simulink model "S13_PASD_as3"  (R2020a)
settings: Solver=VariableStepAuto  StartTime=0.0  StopTime=0.5  RelTol=1e-3
libraries: powerlib x32, cstblocks x1, simulink x1
settings Model: Creator=HP  LastModifiedBy=qm_shail_hash_98
settings DataIOCC: SaveFormat=StructureWithTime  InspectSignalLogs=on  ReturnWorkspaceOutputs=off

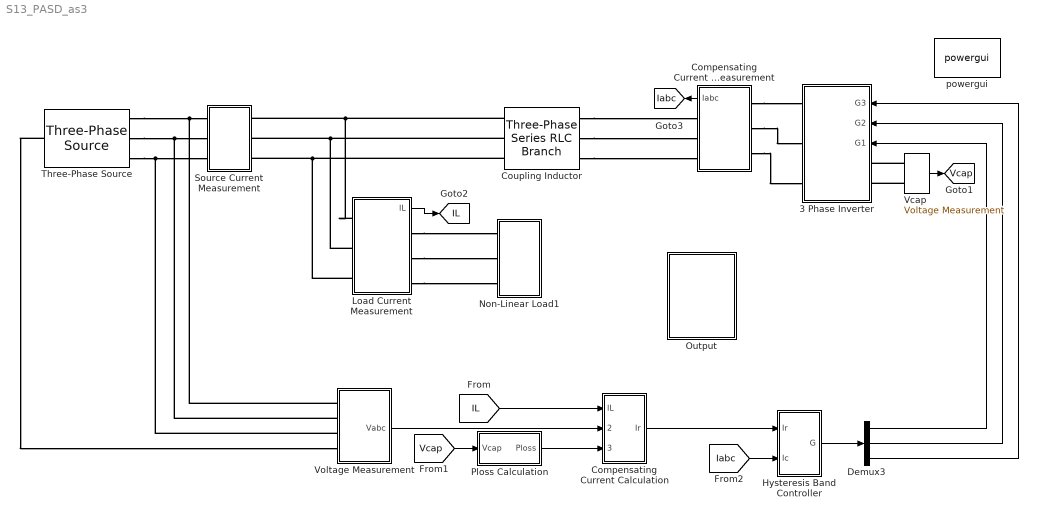
== system S13_PASD_as3 ==
  3 Phase Inverter : Subsystem
  Compensating Current Calculation : Subsystem
  Compensating Current Measurement : Subsystem
  Coupling Inductor : powerlib/Elements/Three-Phase Series RLC Branch  LConnTagsString=A|B|C  RConnTagsString=A|B|C  BranchType=RL  Resistance=0.0001  Inductance=0.0004  Capacitance=1e-6  Measurements=None
  Demux3 : Demux  Outputs=3
  Hysteresis Band Controller : Subsystem
  Load Current Measurement : Subsystem
  "Non-Linear Load1 " : Subsystem
  Output : Subsystem
  Ploss Calculation : Subsystem
  Source Current Measurement : Subsystem
  Three-Phase Source : powerlib/Electrical Sources/Three-Phase Source  InternalConnection=Yn  VoltagePhases=off  Voltage=400  PhaseAngle=0  Voltage_phases=[25e3 25e3 25e3]/sqrt(3)  PhaseAngles_phases=[0 -120 +120]  Frequency=50  NonIdealSource=on  SpecifyImpedance=on  Resistance=0.8929  Inductance=16.58e-3  ShortCircuitLevel=100e6  BaseVoltage=40.83  XRratio=10  BusType=swing  Pref=0  Qref=0  Prefabc=[10e3, 10e3, 10e3]  Qrefabc=[0, 0, 0]  Qmin=-inf  Qmax=inf
  Vcap : powerlib/Measurements/Voltage Measurement  PhasorSimulation=off  OutputType=Complex  PSBequivalent=0
  Voltage Measurement : Subsystem
  powergui : powerlib/powergui  Priority=1  SimulationMode=Discrete  SampleTime=5e-7  frequency=60  Iterations=50  frequencyindice=50  Pbase=100e6  ErrMax=1e-4  UnitsV=kV  UnitsW=MW  buscounter=0  FunctionMessages=off  echomessages=off  EnableUseOfTLC=off  CurrentSourceSwitches=off  DisableSnubberDevices=off  DisableRonSwitches=off  DisableVfSwitches=off  DisplayEquations=off  AutomaticDiscreteSolvers=off  SolverType=Backward Euler  Interpol=off  ExternalGateDelay=off  methode=off  Ts=0  x0status=blocks  SPID=off  SwTol=0  HookPort=off  NonlinearTolerance=1e-4  nMaxIteration=100  ContinueOnMaxIteration=off  RestoreLinks=warning  ResistiveCurrentMeasurement=off  Frange=[0:2:500]  Ylog=off  Xlog=on  ShowGrid=off  save=off  variable=ZData  structure=IS  ZoomFFT=off  StartTime=0.3  cycles=5  DisplayStyle=1  fundamental=50  FreqAxis=off  MaxFrequency=1000  frequencyindicesteady=1  RmsSteady=1  display=off
  tag scope: IL=global, Iabc=global, Vcap=global
  wires:
  Load Current Measurement/1(IL) -> [IL]
  [IL] -> Compensating Current Calculation/1(IL)
  Voltage Measurement/1(Vabc) -> Compensating Current Calculation/2(Vabc)
  Ploss Calculation/1(Ploss) -> Compensating Current Calculation/3(Ploss)
  [Vcap] -> Ploss Calculation/1(Vcap)
  Vcap/1 -> [Vcap]
  Hysteresis Band Controller/1(G) -> Demux3/1
  Demux3/2 -> 3 Phase Inverter/2(G2)
  Compensating Current Calculation/1(Ir) -> Hysteresis Band Controller/1(Ir)
  Compensating Current Measurement/1(Iabc) -> [Iabc]
  [Iabc] -> Hysteresis Band Controller/2(Ic)
  Demux3/1 -> 3 Phase Inverter/3(G1)
  Demux3/3 -> 3 Phase Inverter/1(G3)
  connections:
  Three-Phase Source/RConn1 -- Voltage Measurement/LConn1 -- Source Current Measurement/LConn1
  Three-Phase Source/RConn2 -- Voltage Measurement/LConn2 -- Source Current Measurement/LConn2
  Three-Phase Source/RConn3 -- Voltage Measurement/LConn3 -- Source Current Measurement/LConn3
  Three-Phase Source/LConn1 -- Voltage Measurement/LConn4
  Load Current Measurement/LConn3 -- Coupling Inductor/LConn3 -- Source Current Measurement/RConn3
  Load Current Measurement/LConn1 -- Source Current Measurement/RConn1 -- Coupling Inductor/LConn1
  Load Current Measurement/LConn2 -- Coupling Inductor/LConn2 -- Source Current Measurement/RConn2
  Vcap/LConn2 -- 3 Phase Inverter/LConn2
  Load Current Measurement/RConn1 -- "Non-Linear Load1 "/LConn1
  Load Current Measurement/RConn2 -- "Non-Linear Load1 "/LConn2
  Load Current Measurement/RConn3 -- "Non-Linear Load1 "/LConn3
  Vcap/LConn1 -- 3 Phase Inverter/LConn1
  Compensating Current Measurement/LConn1 -- 3 Phase Inverter/RConn1
  Compensating Current Measurement/LConn2 -- 3 Phase Inverter/RConn2
  Compensating Current Measurement/LConn3 -- 3 Phase Inverter/RConn3
  Coupling Inductor/RConn1 -- Compensating Current Measurement/RConn1
  Coupling Inductor/RConn2 -- Compensating Current Measurement/RConn2
  Coupling Inductor/RConn3 -- Compensating Current Measurement/RConn3

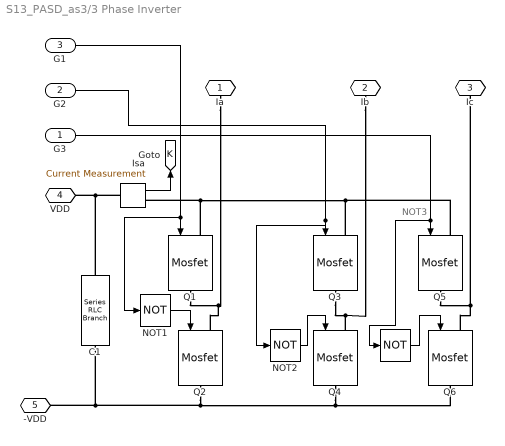
== system S13_PASD_as3/3 Phase Inverter ==
  note: NOT3
  G3 : Inport
  G2 : Inport  Port=2
  G1 : Inport  Port=3
  " " : Logic  Operator=NOT  AllPortsSameDT=off  OutDataTypeStr=boolean
  C1 : powerlib/Elements/Series RLC Branch  LConnTagsString=__new0  RConnTagsString=__new0  BranchType=C  Resistance=1  Inductance=1e-3  SetiL0=off  InitialCurrent=0  Capacitance=500e-6  Setx0=off  InitialVoltage=700  Measurements=None
  Isa : powerlib/Measurements/Current Measurement  PhasorSimulation=off  OutputType=Complex  PSBequivalent=0
  NOT1 : Logic  Operator=NOT  AllPortsSameDT=off  OutDataTypeStr=boolean
  NOT2 : Logic  Operator=NOT  AllPortsSameDT=off  OutDataTypeStr=boolean
  Q{1..6} (6 alike) : powerlib/Power Electronics/Mosfet  Ron=0.01  Lon=0  Rd=0.01  Vfd=0  IC=0  Rs=1e10  Cs=inf  Measurements=off
  Ia : PMIOPort  Side=Right
  Ib : PMIOPort  Port=2  Side=Right
  Ic : PMIOPort  Port=3  Side=Right
  VDD : PMIOPort  Port=4  Side=Left
  -VDD : PMIOPort  Port=5  Side=Left
  tag scope: K=global
  wires:
  NOT1/1 -> Q2/1
  NOT2/1 -> Q4/1
  " "/1 -> Q6/1
  G1/1 -> NOT1/1, Q1/1
  G2/1 -> Q3/1, NOT2/1
  G3/1 -> Q5/1, " "/1
  Isa/1 -> [K]
  connections:
  Q1/RConn1 -- Ia/RConn1 -- Q2/LConn1
  Isa/LConn1 -- VDD/RConn1 -- C1/LConn1
  Q3/RConn1 -- Ib/RConn1 -- Q4/LConn1
  Q6/LConn1 -- Ic/RConn1 -- Q5/RConn1
  Q1/LConn1 -- Isa/RConn1 -- Q5/LConn1 -- Q3/LConn1
  Q2/RConn1 -- C1/RConn1 -- -VDD/RConn1 -- Q4/RConn1 -- Q6/RConn1

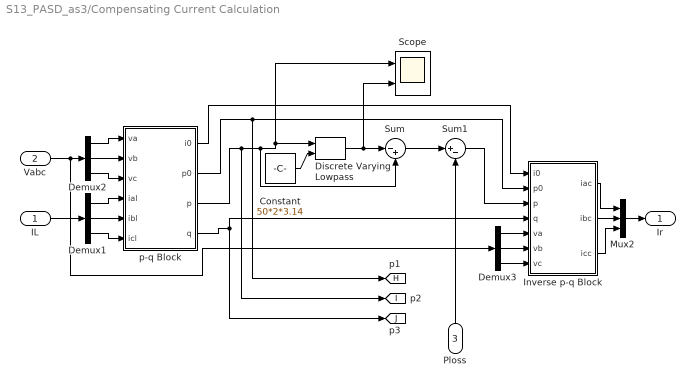
== system S13_PASD_as3/Compensating Current Calculation ==
  IL : Inport
  Vabc : Inport  Port=2
  Ploss : Inport  Port=3
  Constant : Constant  Value=50*2*3.14
  Demux1 : Demux  Outputs=3
  Demux2 : Demux  Outputs=3
  Demux3 : Demux  Outputs=3
  Discrete Varying Lowpass : cstblocks/Linear Parameter Varying/Discrete Varying Lowpass  N=3  w0=0  Ts=1e-3
      settings: SourceProductBaseCode=CT
  Inverse p-q Block : MATLAB Function  TreatAsAtomicUnit=on
  Mux2 : Mux  Inputs=3
  Scope : Scope  NumInputPorts=2
  Sum : Sum  Inputs=|-+
  Sum1 : Sum  Inputs=|+-
  p-q Block : MATLAB Function  TreatAsAtomicUnit=on
  Ir : Outport
  tag scope: H=global, I=global, J=global
  wires:
  Inverse p-q Block/3(icc) -> Mux2/3
  IL/1 -> Demux1/1
  Demux1/2 -> p-q Block/5(ibl)
  Mux2/1 -> Ir/1
  Inverse p-q Block/1(iac) -> Mux2/1
  Demux1/1 -> p-q Block/4(ial)
  Inverse p-q Block/2(ibc) -> Mux2/2
  p-q Block/1(i0) -> Inverse p-q Block/1(i0)
  p-q Block/3(p) -> [I], Scope/1, Discrete Varying Lowpass/1, Sum/2
  Ploss/1 -> Sum1/2
  Discrete Varying Lowpass/1 -> Scope/2, Sum/1
  Sum/1 -> Sum1/1
  Sum1/1 -> Inverse p-q Block/3(p)
  p-q Block/4(q) -> [J], Inverse p-q Block/4(q)
  Demux1/3 -> p-q Block/6(icl)
  p-q Block/2(p0) -> [H], Inverse p-q Block/2(p0)
  Demux2/3 -> p-q Block/3(vc)
  Demux2/2 -> p-q Block/2(vb)
  Demux2/1 -> p-q Block/1(va)
  Vabc/1 -> Demux3/1, Demux2/1
  Demux3/1 -> Inverse p-q Block/5(va)
  Demux3/2 -> Inverse p-q Block/6(vb)
  Demux3/3 -> Inverse p-q Block/7(vc)
  Constant/1 -> Discrete Varying Lowpass/2

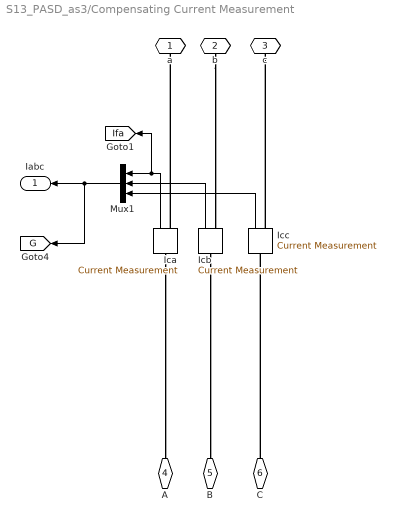
== system S13_PASD_as3/Compensating Current Measurement ==
  Ica : powerlib/Measurements/Current Measurement  PhasorSimulation=off  OutputType=Complex  PSBequivalent=0
  Icb : powerlib/Measurements/Current Measurement  PhasorSimulation=off  OutputType=Complex  PSBequivalent=0
  Icc : powerlib/Measurements/Current Measurement  PhasorSimulation=off  OutputType=Complex  PSBequivalent=0
  Mux1 : Mux  Inputs=3
  a : PMIOPort  Side=Right
  b : PMIOPort  Port=2  Side=Right
  c : PMIOPort  Port=3  Side=Right
  A : PMIOPort  Port=4  Side=Left
  B : PMIOPort  Port=5  Side=Left
  C : PMIOPort  Port=6  Side=Left
  Iabc : Outport
  tag scope: G=global, Ifa=global
  wires:
  Mux1/1 -> [G], Iabc/1
  Ica/1 -> Mux1/1, [Ifa]
  Icc/1 -> Mux1/3
  Icb/1 -> Mux1/2
  connections:
  b/RConn1 -- Icb/RConn1
  Ica/RConn1 -- a/RConn1
  Icc/RConn1 -- c/RConn1
  C/RConn1 -- Icc/LConn1
  Ica/LConn1 -- A/RConn1
  Icb/LConn1 -- B/RConn1

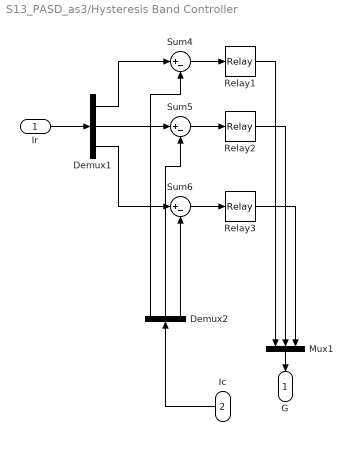
== system S13_PASD_as3/Hysteresis Band Controller ==
  Ir : Inport
  Ic : Inport  Port=2
  Demux1 : Demux  Outputs=3
  Demux2 : Demux  Outputs=3
  Mux1 : Mux  Inputs=3
  Relay1 : Relay  OnSwitchValue=0.0001  OffSwitchValue=-0.0001  ZeroCross=off
  Relay2 : Relay  OnSwitchValue=0.0001  OffSwitchValue=-0.0001  ZeroCross=off
  Relay3 : Relay  OnSwitchValue=0.0001  OffSwitchValue=-0.0001  ZeroCross=off
  Sum4 : Sum  Inputs=|+-
  Sum5 : Sum  Inputs=|+-
  Sum6 : Sum  Inputs=|+-
  G : Outport
  wires:
  Relay3/1 -> Mux1/3
  Relay1/1 -> Mux1/1
  Relay2/1 -> Mux1/2
  Demux2/2 -> Sum5/2
  Demux1/2 -> Sum5/1
  Sum6/1 -> Relay3/1
  Demux1/1 -> Sum4/1
  Demux1/3 -> Sum6/1
  Demux2/3 -> Sum6/2
  Sum5/1 -> Relay2/1
  Demux2/1 -> Sum4/2
  Sum4/1 -> Relay1/1
  Mux1/1 -> G/1
  Ir/1 -> Demux1/1
  Ic/1 -> Demux2/1

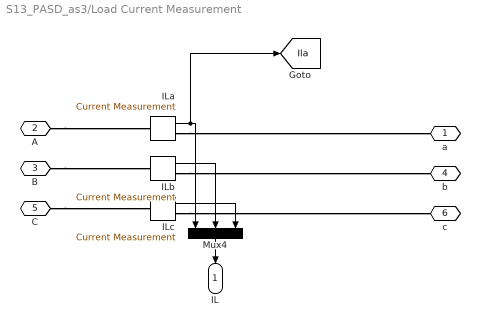
== system S13_PASD_as3/Load Current Measurement ==
  ILa : powerlib/Measurements/Current Measurement  PhasorSimulation=off  OutputType=Complex  PSBequivalent=0
  ILb : powerlib/Measurements/Current Measurement  PhasorSimulation=off  OutputType=Complex  PSBequivalent=0
  ILc : powerlib/Measurements/Current Measurement  PhasorSimulation=off  OutputType=Complex  PSBequivalent=0
  Mux4 : Mux  Inputs=3
  a : PMIOPort  Side=Right
  A : PMIOPort  Port=2  Side=Left
  B : PMIOPort  Port=3  Side=Left
  b : PMIOPort  Port=4  Side=Right
  C : PMIOPort  Port=5  Side=Left
  c : PMIOPort  Port=6  Side=Right
  IL : Outport
  tag scope: Ila=global
  wires:
  Mux4/1 -> IL/1
  ILa/1 -> [Ila], Mux4/1
  ILc/1 -> Mux4/3
  ILb/1 -> Mux4/2
  connections:
  ILb/RConn1 -- b/RConn1
  ILa/RConn1 -- a/RConn1
  ILc/RConn1 -- c/RConn1
  A/RConn1 -- ILa/LConn1
  C/RConn1 -- ILc/LConn1
  B/RConn1 -- ILb/LConn1

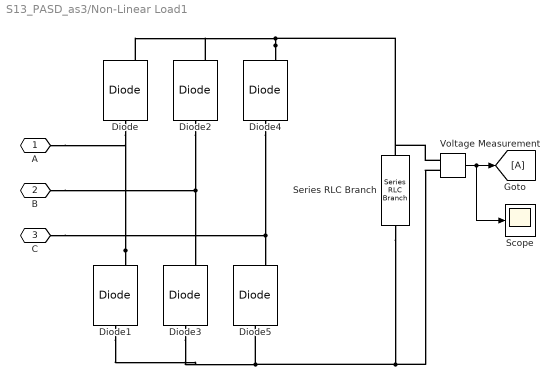
== system S13_PASD_as3/Non-Linear Load1  ==
  Diode{,1..5} (6 alike) : powerlib/Power Electronics/Diode  Ron=0.001  Lon=0  Vf=0.8  IC=0  UseSnubber=0  Rs=500  Cs=250e-9  Measurements=on
  Scope : Scope
  Series RLC Branch : powerlib/Elements/Series RLC Branch  LConnTagsString=__new0  RConnTagsString=__new0  BranchType=RL  Resistance=40  Inductance=0.5  SetiL0=off  InitialCurrent=0  Capacitance=1e-6  Setx0=off  InitialVoltage=0  Measurements=None
  Voltage Measurement : powerlib/Measurements/Voltage Measurement  PhasorSimulation=off  OutputType=Complex  PSBequivalent=0
  A : PMIOPort  Side=Left
  B : PMIOPort  Port=2  Side=Left
  C : PMIOPort  Port=3  Side=Left
  wires:
  Voltage Measurement/1 -> Scope/1, [A]
  connections:
  Diode4/RConn1 -- Voltage Measurement/LConn1 -- Series RLC Branch/LConn1 -- Diode/RConn1 -- Diode2/RConn1
  Series RLC Branch/RConn1 -- Diode5/LConn1 -- Diode1/LConn1 -- Diode3/LConn1 -- Voltage Measurement/LConn2
  Diode1/RConn1 -- Diode/LConn1 -- A/RConn1
  Diode2/LConn1 -- Diode3/RConn1 -- B/RConn1
  Diode4/LConn1 -- C/RConn1 -- Diode5/RConn1

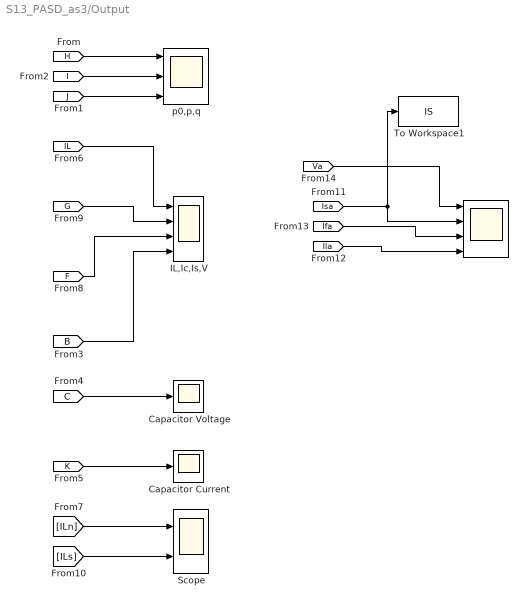
== system S13_PASD_as3/Output ==
  " " : Scope  NumInputPorts=4
  Capacitor Current : Scope
  Capacitor Voltage : Scope
  IL,Ic,Is,V : Scope  NumInputPorts=4
  Scope : Scope  NumInputPorts=2
  To Workspace1 : ToWorkspace  VariableName=IS  SaveFormat=Structure With Time  SampleTime=-1
  p0,p,q : Scope  NumInputPorts=3
  wires:
  [C] -> Capacitor Voltage/1
  [F] -> IL,Ic,Is,V/3
  [IL] -> IL,Ic,Is,V/1
  [B] -> IL,Ic,Is,V/4
  [G] -> IL,Ic,Is,V/2
  [H] -> p0,p,q/1
  [I] -> p0,p,q/2
  [J] -> p0,p,q/3
  [K] -> Capacitor Current/1
  [ILn] -> Scope/1
  [ILs] -> Scope/2
  [Ila] -> " "/4
  [Ifa] -> " "/3
  [Isa] -> To Workspace1/1, " "/2
  [Va] -> " "/1

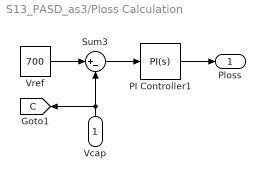
== system S13_PASD_as3/Ploss Calculation ==
  Vcap : Inport
  PI Controller1 : simulink/Continuous/PID Controller  Controller=PI  Form=Parallel  TimeDomain=Continuous-time  UseExternalTs=off  SampleTime=-1  IntegratorMethod=Forward Euler  FilterMethod=Forward Euler  ControllerParametersSource=internal  P=31.1  I=5  D=0  UseFilter=on  N=100  TunerSelectOption=Frequency Response Based  ZeroCross=off  InitialConditionSource=internal  InitialConditionForIntegrator=0  InitialConditionForFilter=0  DifferentiatorICPrevScaledInput=0  ExternalReset=none  TrackingMode=off  Kt=1  LimitOutput=off  UpperSaturationLimit=inf  LowerSaturationLimit=-inf  LinearizeAsGain=off  AntiWindupMode=none  Kb=1  POutMin=[]  POutMax=[]  IOutMin=[]  IOutMax=[]  DOutMin=[]  DOutMax=[]  NOutMin=[]  NOutMax=[]  SumOutMin=[]  SumOutMax=[]  SaturationOutMin=[]  SaturationOutMax=[]  PParamMin=[]  PParamMax=[]  IParamMin=[]  IParamMax=[]  DParamMin=[]  DParamMax=[]  NParamMin=[]  NParamMax=[]  KbParamMin=[]  KbParamMax=[]  KtParamMin=[]  KtParamMax=[]  KbOutMin=[]  KbOutMax=[]  KtOutMin=[]  KtOutMax=[]  IntegratorOutMin=[]  IntegratorOutMax=[]  FilterOutMin=[]  FilterOutMax=[]  SumI1OutMin=[]  SumI1OutMax=[]  SumI2OutMin=[]  SumI2OutMax=[]  SumI3OutMin=[]  SumI3OutMax=[]  SumI4OutMin=[]  SumI4OutMax=[]  SumDOutMin=[]  SumDOutMax=[]  DifferentiatorOutMin=[]  DifferentiatorOutMax=[]  FilterDiffOutCoefMin=[]  FilterDiffOutCoefMax=[]  ReciprocalOutMin=[]  ReciprocalOutMax=[]  SumDenOutMin=[]  SumDenOutMax=[]  SumNumOutMin=[]  SumNumOutMax=[]  DivideOutMin=[]  DivideOutMax=[]  UdiffTsProdOutMin=[]  UdiffTsProdOutMax=[]  NTsProdOutMin=[]  NTsProdOutMax=[]  UintegralTsProdOutMin=[]  UintegralTsProdOutMax=[]  UngainTsProdOutMin=[]  UngainTsProdOutMax=[]  IntegratorContinuousStateAttributes=''  IntegratorStateMustResolveToSignalObject=off  IntegratorRTWStateStorageClass=Auto  FilterContinuousStateAttributes=''  FilterStateMustResolveToSignalObject=off  FilterRTWStateStorageClass=Auto  ParallelPVariant=InternalParameters  IdealPVariant=Disabled  IVariant=InternalParameters  DVariant=Disabled  IntegratorVariant=Continuous  SatVariant=Disabled  AWVariant=Passthrough  PCopyVariant=Disabled  TRVariant=Disabled  FdbkBlocksVariant=Forward  IdealPFdbkVariant=Disabled  SatFdbkVariant=Disabled  DerivativeFilterVariant=Disabled  NVariant=Disabled  NCopyVariant=Disabled_SignalSpec  FilterICVariant=Disabled  IntegratorICVariant=InternalICs  ExternalResetVariant=Disabled  TRSumVariant=Passthrough  SumFdbkVariant=Disabled  SumVariant=Sum_PI  TsampFilterVariant=InternalTs  TsampNgainVariant=Passthrough  TsampIntegralVariant=Passthrough
  Sum3 : Sum  Inputs=|+-
  Vref : Constant  Value=700
  Ploss : Outport
  tag scope: C=global
  wires:
  Vcap/1 -> Sum3/2, [C]
  Vref/1 -> Sum3/1
  Sum3/1 -> PI Controller1/1
  PI Controller1/1 -> Ploss/1

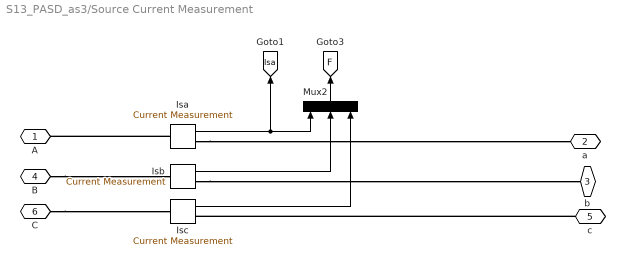
== system S13_PASD_as3/Source Current Measurement ==
  Isa : powerlib/Measurements/Current Measurement  PhasorSimulation=off  OutputType=Complex  PSBequivalent=0
  Isb : powerlib/Measurements/Current Measurement  PhasorSimulation=off  OutputType=Complex  PSBequivalent=0
  Isc : powerlib/Measurements/Current Measurement  PhasorSimulation=off  OutputType=Complex  PSBequivalent=0
  Mux2 : Mux  Inputs=3
  A : PMIOPort  Side=Left
  a : PMIOPort  Port=2  Side=Right
  b : PMIOPort  Port=3  Side=Right
  B : PMIOPort  Port=4  Side=Left
  c : PMIOPort  Port=5  Side=Right
  C : PMIOPort  Port=6  Side=Left
  tag scope: F=global, Isa=global
  wires:
  Isc/1 -> Mux2/3
  Isb/1 -> Mux2/2
  Isa/1 -> [Isa], Mux2/1
  Mux2/1 -> [F]
  connections:
  Isa/RConn1 -- a/RConn1
  B/RConn1 -- Isb/LConn1
  Isb/RConn1 -- b/RConn1
  c/RConn1 -- Isc/RConn1
  C/RConn1 -- Isc/LConn1
  Isa/LConn1 -- A/RConn1

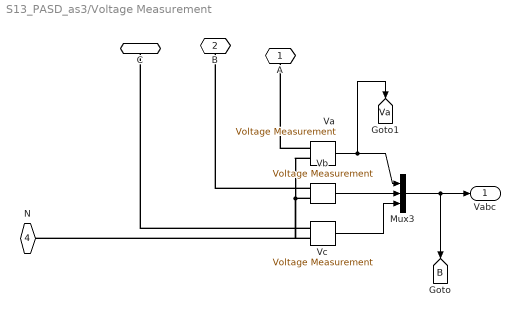
== system S13_PASD_as3/Voltage Measurement ==
  Mux3 : Mux  Inputs=3
  Va : powerlib/Measurements/Voltage Measurement  PhasorSimulation=off  OutputType=Complex  PSBequivalent=0
  Vb : powerlib/Measurements/Voltage Measurement  PhasorSimulation=off  OutputType=Complex  PSBequivalent=0
  Vc : powerlib/Measurements/Voltage Measurement  PhasorSimulation=off  OutputType=Complex  PSBequivalent=0
  A : PMIOPort  Side=Left
  B : PMIOPort  Port=2  Side=Left
  C : PMIOPort  Port=3  Side=Left
  N : PMIOPort  Port=4  Side=Left
  Vabc : Outport
  tag scope: B=global, Va=global
  wires:
  Mux3/1 -> [B], Vabc/1
  Vc/1 -> Mux3/3
  Vb/1 -> Mux3/2
  Va/1 -> [Va], Mux3/1
  connections:
  Vc/LConn1 -- C/RConn1
  Vb/LConn1 -- B/RConn1
  Va/LConn1 -- A/RConn1
  Va/LConn2 -- Vc/LConn2 -- N/RConn1 -- Vb/LConn2

== matlab function S13_PASD_as3/Compensating Current Calculation/Inverse p-q Block ==
  data: i0 input; p0 input; p input; iac output; q input; va input; vb input; vc input; ibc output; icc output
function [iac,ibc,icc]= fcn(i0,p0,p,q,va,vb,vc)
%#codegen
v_zero=(va+vb+vc)/sqrt(3);
v_alpha=(va-vb/2-vc/2)*sqrt(2/3);
v_beta=(vb-vc)/sqrt(2);
i_zero=i0;
i_alpha=(v_alpha.*p+v_beta.*q)/(v_alpha.^2+v_beta.^2);
i_beta=(v_beta.*p-v_alpha.*q)/(v_alpha.^2+v_beta.^2);
iac=sqrt(2/3)*(i_zero/sqrt(2)+i_alpha);
ibc=sqrt(2/3)*(i_zero./sqrt(2)-i_alpha/2+sqrt(3)*i_beta/2);
icc=sqrt(2/3)*(i_zero./sqrt(2)-i_alpha/2-i_beta*sqrt(3)/2);

== matlab function S13_PASD_as3/Compensating Current Calculation/p-q Block ==
  data: i0 output; p0 output; va input; p output; vb input; vc input; ial input; ibl input; icl input; q output
function [i0,p0,p,q]= fcn(va,vb,vc,ial,ibl,icl)
%#codegen
v_zero=(va+vb+vc)/sqrt(3);
v_alpha=(va-vb/2-vc/2)*sqrt(2/3);
v_beta=(vb-vc)/sqrt(2);
il_zero=(ial+ibl+icl)/sqrt(3);
il_alpha=(ial-ibl/2-icl/2)*sqrt(2/3);
il_beta=(ibl-icl)/sqrt(2);
i0=il_zero;
p0=v_zero.*il_zero;
p=v_alpha.*il_alpha+v_beta.*il_beta;
q=v_beta.*il_alpha-v_alpha.*il_beta;
